simulink model "sldemo_mdlref_bus"  (Simulink 10.0)
settings: Solver=FixedStepDiscrete  StartTime=0.0  StopTime=30  FixedStep=0.1  RelTol=1e-3  EnableMultiTasking=on
PreLoadFcn:
  | load sldemo_mdlref_counter_bus.mat
libraries: SignalEditorBlockLib x1
settings Model: Creator=The MathWorks, Inc.  ModifiedByFormat=The MathWorks Inc.  LastModifiedBy=The MathWorks Inc.  ExtModeAutoUpdateStatusClock=off
settings DataIOCC: SaveFormat=Dataset  SaveOutput=off  SaveTime=off  SignalLoggingName=topOut
settings OptimizationCC: DefaultParameterBehavior=Inlined  InlineInvariantSignals=on  ExpressionDepthLimit=2147483647  InitFltsAndDblsToZero=on
settings DebuggingCC: SaveWithParameterizedLinksMsg=none  UnderspecifiedInitializationDetection=Simplified  MergeDetectMultiDrivingBlocksExec=error  CheckExecutionContextPreStartOutputMsg=on  CheckExecutionContextRuntimeOutputMsg=on  MultiTaskDSMMsg=warning  MultiTaskCondExecSysMsg=none  SigSpecEnsureSampleTimeMsg=none  FcnCallInpInsideContextMsg=warning  BusObjectLabelMismatch=error  AllowSymbolicDim=off  ModelReferenceDataLoggingMessage=none  StateNameClashWarn=warning  StrictBusMsg=ErrorOnBusTreatedAsVector
settings HardwareCC: TargetHWDeviceType=32-bit Generic
settings ModelReferenceCC: UpdateModelReferenceTargets=IfOutOfDate
settings RTWCC: GenerateReport=on  LaunchReport=on
settings CodeAppCC: MaxIdLength=100
settings GRTTargetCC: TargetFcnLib=ansi_tfl_tmw.mat  GeneratePreprocessorConditionals=Disable all  MatFileLogging=off
settings ConfigComp: CovExternalEMLEnable=off  CovSFcnEnable=off

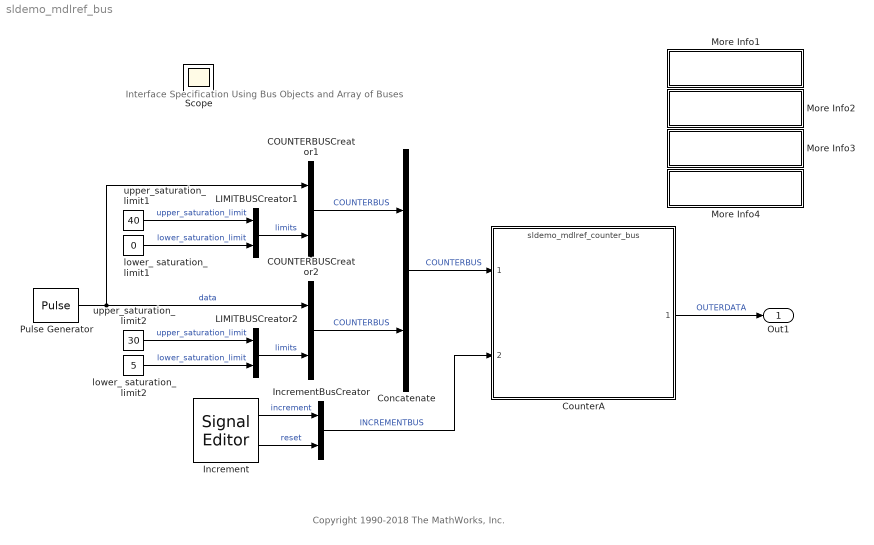
== system sldemo_mdlref_bus ==
  note: Interface Specification Using Bus Objects and Array of Buses
  note: Copyright 1990-2018 The MathWorks, Inc.
  COUNTERBUSCreator1 : BusCreator  Inputs=2  OutDataTypeStr=Bus: COUNTERBUS  NonVirtualBus=on
  COUNTERBUSCreator2 : BusCreator  Inputs=2  OutDataTypeStr=Bus: COUNTERBUS  NonVirtualBus=on
  Concatenate : Concatenate  Mode=Multidimensional array
  CounterA : ModelReference  ModelNameDialog=sldemo_mdlref_counter_bus  SimulationMode=Normal  ModelReferenceVersion=1.272
  Increment : SignalEditorBlockLib/Signal Editor  FileName=sldemo_mdlref_bus_data.mat  ActiveScenario=Group1  ActiveSignal=Reset  IsBus=off  OutputBusObjectStr=Bus: BusObject  SampleTime=0.1  OutputAfterFinalValue=Holding final value  Unit=inherit  PreserveSignalName=on
      settings: SourceProductName=Simulink
  IncrementBusCreator : BusCreator  Inputs=2  OutDataTypeStr=Bus: INCREMENTBUS  NonVirtualBus=on
  LIMITBUSCreator1 : BusCreator  Inputs=2  OutDataTypeStr=Bus: LIMITBUS  NonVirtualBus=on
  LIMITBUSCreator2 : BusCreator  Inputs=2  OutDataTypeStr=Bus: LIMITBUS  NonVirtualBus=on
  More Info1 : Subsystem
      settings: OpenFcn=helpview(fullfile(docroot,'simulink','helptargets.map'),'sldemo_mdlref_bus')
      mask Display: disp('Interface Specification')
  More Info2 : Subsystem
      settings: OpenFcn=helpview(fullfile(docroot,'simulink','helptargets.map'),'sldemo_mdlref_protect')
      mask Display: disp('Protected Models')
  More Info3 : Subsystem
      settings: OpenFcn=helpview(fullfile(docroot,'simulink','helptargets.map'),'sldemo_mdlref_logging_intervals')
      mask Display: disp('Logging Intervals')
  More Info4 : Subsystem
      settings: OpenFcn=helpview(fullfile(docroot,'simulink','helptargets.map'),'sldemo_working_with_big_data')
      mask Display: disp('Working with Big Data')
  Pulse Generator : DiscretePulseGenerator  Amplitude=int32(1)  SampleTime=0.1
  lower_ saturation_ limit1 : Constant  Value=0  OutDataTypeStr=int32
  lower_ saturation_ limit2 : Constant  Value=5  OutDataTypeStr=int32
  upper_saturation_limit1 : Constant  Value=40  OutDataTypeStr=int32
  upper_saturation_limit2 : Constant  Value=30  OutDataTypeStr=int32
  Out1 : Outport  VectorParamsAs1DForOutWhenUnconnected=off
  Scope : Scope
  wires:
  Concatenate/1 -> CounterA/1  "COUNTERBUS"
  CounterA/1 -> Out1/1  "OUTERDATA"
  Increment/1 -> IncrementBusCreator/1  "increment"
  Increment/2 -> IncrementBusCreator/2  "reset"
  IncrementBusCreator/1 -> CounterA/2  "INCREMENTBUS"
  COUNTERBUSCreator1/1 -> Concatenate/1  "COUNTERBUS"
  LIMITBUSCreator1/1 -> COUNTERBUSCreator1/2  "limits"
  COUNTERBUSCreator2/1 -> Concatenate/2  "COUNTERBUS"
  LIMITBUSCreator2/1 -> COUNTERBUSCreator2/2  "limits"
  upper_saturation_limit1/1 -> LIMITBUSCreator1/1  "upper_saturation_limit"
  lower_ saturation_ limit1/1 -> LIMITBUSCreator1/2  "lower_saturation_limit"
  Pulse Generator/1 -> COUNTERBUSCreator1/1, COUNTERBUSCreator2/1  "data"
  upper_saturation_limit2/1 -> LIMITBUSCreator2/1  "upper_saturation_limit"
  lower_ saturation_ limit2/1 -> LIMITBUSCreator2/2  "lower_saturation_limit"

== system sldemo_mdlref_bus/More Info1 ==
  note: This demonstration shows how signals may be grouped and ungrouped while
      | retaining their names.  In this demonstration, 5 signals are created and labeled
      | appropriately.  These signals are then grouped together to create a bus of signals.
      | This bus of signals is then fed into the Bus Selector block.  Inside of the Bus
      | Selector block, the Pulse and Chirp signals are chosen to be output from the
      | original signal bus.
      |
      | It is possible to place a nest signal buses and then still retrieve the original signal
      | with its label.
  note: Bus Block Demonstration

== system sldemo_mdlref_bus/More Info2 ==
  note: Bus Block Demonstration
  note: This demonstration shows how signals may be grouped and ungrouped while
      | retaining their names.  In this demonstration, 5 signals are created and labeled
      | appropriately.  These signals are then grouped together to create a bus of signals.
      | This bus of signals is then fed into the Bus Selector block.  Inside of the Bus
      | Selector block, the Pulse and Chirp signals are chosen to be output from the
      | original signal bus.
      |
      | It is possible to place a nest signal buses and then still retrieve the original signal
      | with its label.

== system sldemo_mdlref_bus/More Info3 ==
  note: This demonstration shows how signals may be grouped and ungrouped while
      | retaining their names.  In this demonstration, 5 signals are created and labeled
      | appropriately.  These signals are then grouped together to create a bus of signals.
      | This bus of signals is then fed into the Bus Selector block.  Inside of the Bus
      | Selector block, the Pulse and Chirp signals are chosen to be output from the
      | original signal bus.
      |
      | It is possible to place a nest signal buses and then still retrieve the original signal
      | with its label.
  note: Bus Block Demonstration

== system sldemo_mdlref_bus/More Info4 ==
  note: Bus Block Demonstration
  note: This demonstration shows how signals may be grouped and ungrouped while
      | retaining their names.  In this demonstration, 5 signals are created and labeled
      | appropriately.  These signals are then grouped together to create a bus of signals.
      | This bus of signals is then fed into the Bus Selector block.  Inside of the Bus
      | Selector block, the Pulse and Chirp signals are chosen to be output from the
      | original signal bus.
      |
      | It is possible to place a nest signal buses and then still retrieve the original signal
      | with its label.
